simulink model "mdl"  (R2022a)
settings: Solver=FixedStepAuto  StartTime=0.0  StopTime=5  FixedStep=1e-5  RelTol=1e-3
libraries: simulink x1
settings Model: Creator=Tsing  LastModifiedBy=Tsing

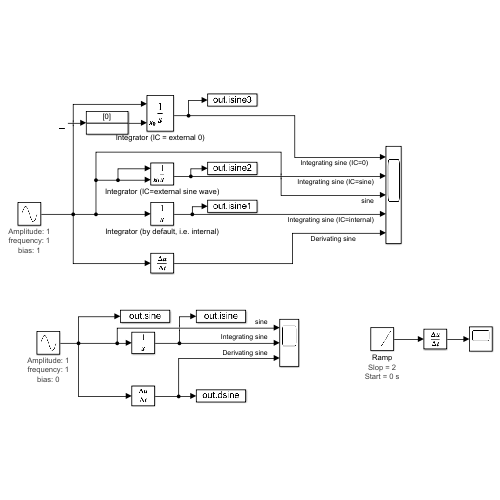
[thumbnail: Simulink's stored preview of the top-level diagram]
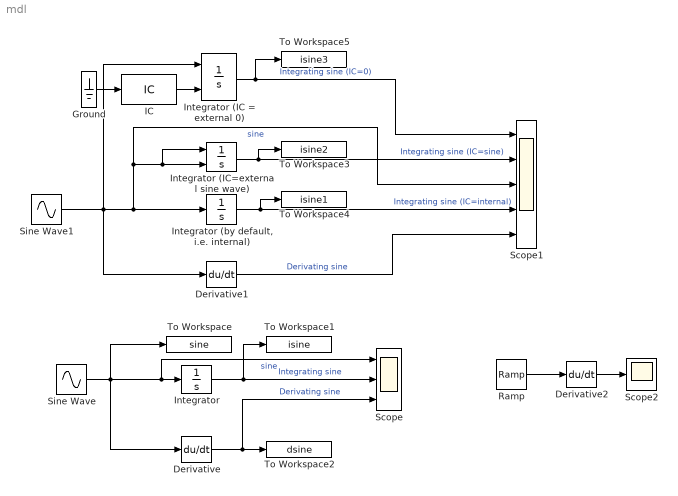
== system mdl ==
  Derivative : Derivative
  Derivative1 : Derivative
  Derivative2 : Derivative
  Ground : Ground
  IC : InitialCondition  Value=0
  Integrator : Integrator
  Integrator (IC = external 0) : Integrator  InitialConditionSource=external  InitialCondition=1
  Integrator (IC=external sine wave) : Integrator  InitialConditionSource=external  InitialCondition=1
  "Integrator (by default, i.e. internal)" : Integrator  InitialCondition=1
  Ramp : simulink/Sources/Ramp  slope=2  start=0  InitialOutput=0
      settings: AttributesFormatString=|
      | Slop = %<slope>
      | Start = %<start> s
  Scope : Scope  NumInputPorts=3
  Scope1 : Scope  NumInputPorts=5
  Scope2 : Scope
  Sine Wave : Sin  SampleTime=0
      settings: AttributesFormatString=|
      | Amplitude: %<Amplitude>
      | frequency: %<Frequency>
      | bias: %<Bias>
  Sine Wave1 : Sin  Bias=1  SampleTime=0
      settings: AttributesFormatString=|
      | Amplitude: %<Amplitude>
      | frequency: %<Frequency>
      | bias: %<Bias>
  To Workspace : ToWorkspace  VariableName=sine  SaveFormat=Timeseries  SampleTime=-1
  To Workspace1 : ToWorkspace  VariableName=isine  SaveFormat=Timeseries  SampleTime=-1
  To Workspace2 : ToWorkspace  VariableName=dsine  SaveFormat=Timeseries  SampleTime=-1
  To Workspace3 : ToWorkspace  VariableName=isine2  SaveFormat=Timeseries  SampleTime=-1
  To Workspace4 : ToWorkspace  VariableName=isine1  SaveFormat=Timeseries  SampleTime=-1
  To Workspace5 : ToWorkspace  VariableName=isine3  SaveFormat=Timeseries  SampleTime=-1
  wires:
  Sine Wave/1 -> To Workspace/1, Derivative/1, Scope/1, Integrator/1  "sine"
  Integrator/1 -> Scope/2, To Workspace1/1  "Integrating sine"
  Derivative/1 -> Scope/3, To Workspace2/1  "Derivating sine"
  Derivative1/1 -> Scope1/5  "Derivating sine"
  "Integrator (by default, i.e. internal)"/1 -> To Workspace4/1, Scope1/4  "Integrating sine (IC=internal)"
  Sine Wave1/1 -> Integrator (IC = external 0)/1, Integrator (IC=external sine wave)/1, Integrator (IC=external sine wave)/2, Scope1/3, "Integrator (by default, i.e. internal)"/1, Derivative1/1  "sine"
  Ramp/1 -> Derivative2/1
  Derivative2/1 -> Scope2/1
  Integrator (IC=external sine wave)/1 -> To Workspace3/1, Scope1/2  "Integrating sine (IC=sine)"
  Ground/1 -> IC/1
  IC/1 -> Integrator (IC = external 0)/2
  Integrator (IC = external 0)/1 -> To Workspace5/1, Scope1/1  "Integrating sine (IC=0)"
